simulink model "Tutorial20"  (R2020a)
settings: Solver=FixedStepDiscrete  StartTime=0.0  StopTime=10.0  FixedStep=1.0  RelTol=1e-3
values from neighbouring files (symbols this model uses):
  Temperature = [0 1 2 3 4 5 6 7 8 9 10 11 ... (101 elements, 101x1)]    [InputData.mat]
  Voltage = [0.5 0.54 0.58 0.62 0.66 0.7 0.74 0.78 0.82 0.86 0.9 0.94 ... (101 elements, 101x1)]    [InputData.mat]
libraries: simulink x2
settings Model: Creator=ashok  LastModifiedBy=ashok

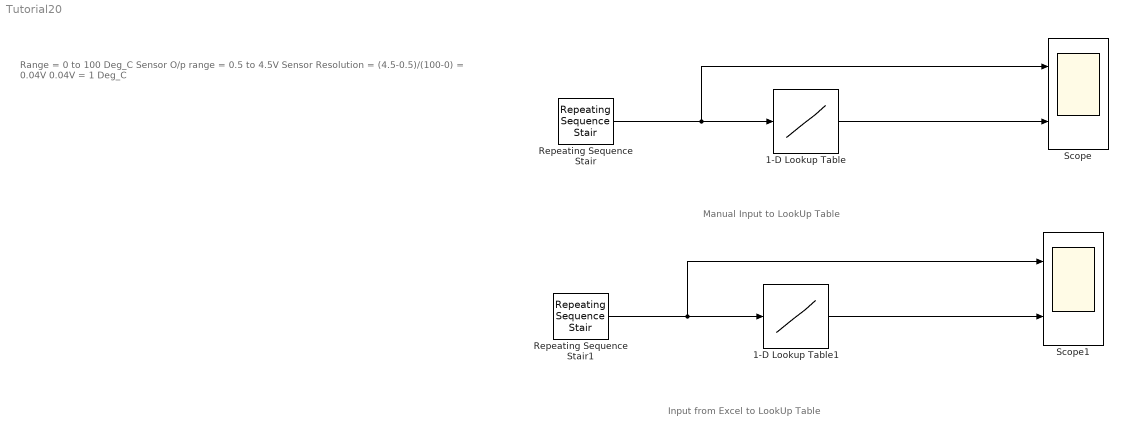
== system Tutorial20 ==
  note: Manual Input to LookUp Table
  note: Range = 0 to 100 Deg_C
      |
      | Sensor O/p range = 0.5 to 4.5V
      |
      | Sensor Resolution = (4.5-0.5)/(100-0) = 0.04V
      |
      | 0.04V = 1 Deg_C
  note: Input from Excel to LookUp Table
  1-D Lookup Table : Lookup_n-D  NumberOfTableDimensions=1  BreakpointsForDimension1=[0.5:0.04:4.5]  Table=[0:1:100]  InternalRulePriority=Speed  RndMeth=Simplest  InputSameDT=on
  1-D Lookup Table1 : Lookup_n-D  NumberOfTableDimensions=1  BreakpointsForDimension1=Voltage  Table=Temperature  InternalRulePriority=Speed  RndMeth=Simplest  InputSameDT=on
  Repeating Sequence Stair : simulink/Sources/Repeating Sequence Stair  OutValues=Sensor_Data  tsamp=-1  OutMin=[]  OutMax=[]  OutDataTypeStr=double  OutputDataTypeScalingMode=double  OutDataType=fixdt(0,8)  ConRadixGroup=Best Precision: Vector-wise  OutScaling=2^-12
  Repeating Sequence Stair1 : simulink/Sources/Repeating Sequence Stair  OutValues=Sensor_Data  tsamp=-1  OutMin=[]  OutMax=[]  OutDataTypeStr=double  OutputDataTypeScalingMode=double  OutDataType=fixdt(0,8)  ConRadixGroup=Best Precision: Vector-wise  OutScaling=2^-12
  Scope : Scope  NumInputPorts=2
  Scope1 : Scope  NumInputPorts=2
  wires:
  Repeating Sequence Stair/1 -> Scope/1, 1-D Lookup Table/1
  Repeating Sequence Stair1/1 -> Scope1/1, 1-D Lookup Table1/1
  1-D Lookup Table1/1 -> Scope1/2
  1-D Lookup Table/1 -> Scope/2
